simulink model "trojpolozeniowy_kor"  (R2018b)
settings: Solver=VariableStepAuto  StartTime=0.0  StopTime=30  RelTol=1e-3
settings Model: Creator=groinder  LastModifiedBy=krzys
settings SolverCC: ZeroCrossAlgorithm=Adaptive
settings DebuggingCC: IgnoredZcDiagnostic=none

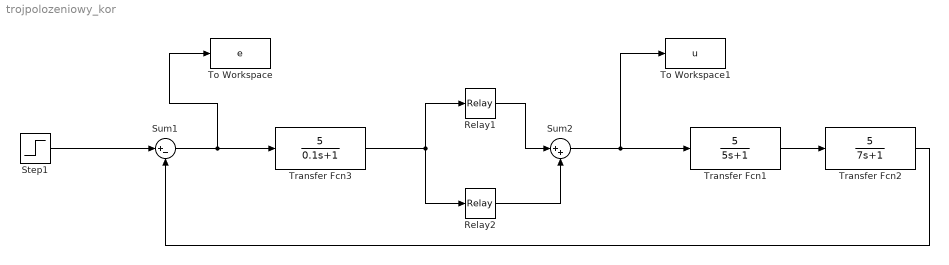
== system trojpolozeniowy_kor ==
  Relay1 : Relay  OnSwitchValue=0.8  OffSwitchValue=-0.6
  Relay2 : Relay  OnSwitchValue=0.6  OffSwitchValue=-0.8  OnOutputValue=0  OffOutputValue=-1
  Step1 : Step  SampleTime=0
  Sum1 : Sum  Inputs=|+-
  Sum2 : Sum  Inputs=|++
  To Workspace : ToWorkspace  VariableName=e  SaveFormat=Structure With Time  SampleTime=-1
  To Workspace1 : ToWorkspace  VariableName=u  SaveFormat=Structure With Time  SampleTime=-1
  Transfer Fcn1 : TransferFcn  Numerator=[5]  Denominator=[5 1]
  Transfer Fcn2 : TransferFcn  Numerator=[5]  Denominator=[7 1]
  Transfer Fcn3 : TransferFcn  Numerator=[5]  Denominator=[0.1 1]
  wires:
  Step1/1 -> Sum1/1
  Transfer Fcn2/1 -> Sum1/2
  Relay2/1 -> Sum2/2
  Relay1/1 -> Sum2/1
  Sum1/1 -> To Workspace/1, Transfer Fcn3/1
  Transfer Fcn1/1 -> Transfer Fcn2/1
  Sum2/1 -> Transfer Fcn1/1, To Workspace1/1
  Transfer Fcn3/1 -> Relay1/1, Relay2/1
